simulink model "EndeVeranstaltungNumet24_01_11"  (R2023b)
settings: Solver=ode1  StartTime=0.0  StopTime=10.0  FixedStep=0.0001  RelTol=1e-3
settings Model: Creator=PM  LastModifiedBy=PM

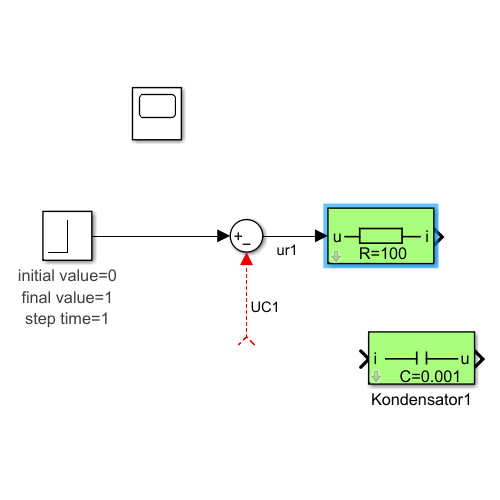
[thumbnail: Simulink's stored preview of the top-level diagram]
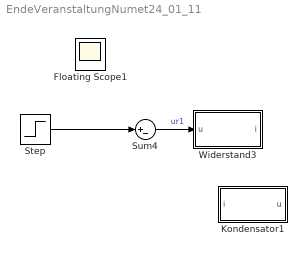
== system EndeVeranstaltungNumet24_01_11 ==
  Floating Scope1 : Scope
      settings: Floating=on
  Kondensator1 : Subsystem  mask{C=1E-3}
      mask prompts: C "Kappazität C [F]"
      mask help:
      | Kapazität
      | Eingang ist u, Ausgang ist i.
      | i=1/C * integral(u)
      mask Display:
      | plot(0,0)
      | plot(100,100)
      | plot([0 0],[1 1]) %Umschalten auf dicke Linien
      | %patch([30 30 70 70 30],[40 60 60 40 40],[0,0,0])
      | plot([45 45],[40 60])
      | plot([55 55],[40 60])
      | plot([15 45],[50 50])
      | 
      | plot([55 85],[50 50])
      | 
      | 
      | 
      | text(30,19,['C=',num2str(C)])
      | 
      | 
      | 
      | port_label ('output',1,'u')
      | port_label ('input',1,'i')
  Step : Step  SampleTime=0
      settings: AttributesFormatString=initial value=%<Before>\nfinal value=%<After>\nstep time=%<Time>
  Sum4 : Sum  Inputs=|+-
  Widerstand3 : Subsystem  mask{R=100}
      mask prompts: R "Widerstand [Ohm]"
      mask help: Ohm'scher Widerstand, Eingang ist u, Ausgang ist i.
      mask Display:
      | plot(0,0)
      | plot(100,100)
      | plot([0 0],[1 1]) %Umschalten auf dicke Linien
      | plot([30 30 70 70 30],[35 65 65 35 35])
      | plot([15 30],[50 50])
      | plot([70 88],[50 50])
      | 
      | 
      | text(30,20,['R=',num2str(R)])
      | 
      | 
      | 
      | port_label ('output',1,'i')
      | port_label ('input',1,'u')
  wires:
  Step/1 -> Sum4/1
  Sum4/1 -> Widerstand3/1(u)  "ur1"
  ? -> Sum4/2  "UC1"

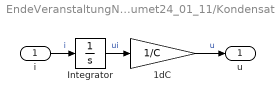
== system EndeVeranstaltungNumet24_01_11/Kondensator1 ==
  i : Inport
  1dC : Gain  Gain=1/C
  Integrator : Integrator
  u : Outport  VectorParamsAs1DForOutWhenUnconnected=off
  wires:
  Integrator/1 -> 1dC/1  "ui"
  1dC/1 -> u/1  "u"
  i/1 -> Integrator/1  "i"

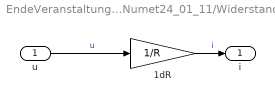
== system EndeVeranstaltungNumet24_01_11/Widerstand3 ==
  u : Inport
  1dR : Gain  Gain=1/R
  i : Outport  VectorParamsAs1DForOutWhenUnconnected=off
  wires:
  1dR/1 -> i/1  "i"
  u/1 -> 1dR/1  "u"
